simulink model "V1_DC_AC_PR_GF"  (R2022b)
settings: Solver=VariableStepAuto  StartTime=0.0  StopTime=.2  RelTol=1e-3
InitFcn:
  | %% Initialize twist parameters
  | source_V = 0;
  | Ts = 1e-7;
  | 
  | % set the PID parameters
  | Kp = 0.000215;
  | Ti = 7.5175e-5;
  | Td = 0.0;
  | N  = 0.0;
  | Kd = 0.0;
  | kp= 0.02;
  | kr = 4000;
  | fr = 10e3;
  | 
  | 
  | %Low side parameters
  | twist_low_side_L = 33e-6;
  | twist_low_side_rL = 20e-3; %Modified
  | twist_low_side_C = 47e-6 + 3*4.7e-6;
  | twist_low_side_C_electrolytic = 47e-6;
  | twist_low_side_C_ceramic = 3*4.7e-6;
  | twist_low_side_rC = 700e-3;
  | twist_low_side_rC_ceramic = 0;
  | twist_low_side_adc_R = 150e3+470;
  | 
  | %High side parameters
  | twist_high_side_C = 33e-6*4 + 4.7e-6*12;
  | twist_high_side_rC = 0.1;
  | twist_high_side_adc_R = 1/(1/2e6 + 1/2e6 + 1/(330e3+5.6e3));
  | twist_high_side_feeder_R = 47e3+4.7e3;
  | R_parallel = 1/(1/twist_high_side_adc_R + 1/twist_high_side_feeder_R);
  | tau_VCC = 0.204;
  | tau_desactive = 0.2;
  | twist_R_VCC = (tau_VCC/twist_high_side_C  - twist_high_side_rC)/(1-(tau_VCC/twist_high_side_C - twist_high_side_rC)/R_parallel);
  | 
  | %High side feeder current
  | %load('feeder_current.mat');
  | feeder_VHigh_min = 12;
  | feeder_VHigh_spacing = 6;
  | feeder_duty_min = 0.1;
  | feeder_duty_spacing = 0.4;
  | feeder_Vth_stop = 8.9;
  | feeder_Vth_start = 9.7;
  | feeder_current_upper_rate_limit = 0.386/(20e-3);
  | feeder_current_lower_rate_limit = -500;
  | 
  | %MOSFET parameters
  | twist_FET_Ron = 0.016;
  | twist_FET_Lon = 0;
  | twist_FET_Rd = 0.006;
  | twist_FET_Vf = 0.7;
  | twist_FET_Rs = 1e10;
  | twist_FET_Cs = inf;
  | twist_FET_Clow_Ron = 220e-3;
  | twist_FET_Clow_Rd = 45e-3; %Modified
  | twist_FET_Clow_Vf = 0.7; %Modified
  | 
  | 
  | %Schottky diode parameters
  | twist_shottky_Ron = 0.48; %Modified
  | twist_shottky_Vf = 0.28; %Modified
  | twist_shottky_Rs = 1e10;
  | twist_shottky_Cs = inf;
  | 
  | %PWM generation
  | twist_freq_switching = 200e3; %carry switching frequency
  | twist_period_switching = 1/twist_freq_switching; %carry switching period
  | twist_pwm_resolution = 100e-9; %resolution of the PWM generator - increasing it reduces simulation time
  | twist_duty_cycle_min = 0; %minimum duty cycle
  | twist_duty_cycle_max = 1; %maximum duty cycle
  | twist_dead_time = 200e-9; %duty cycle positive dead time
  | 
  | % Initialize times and frequencies
  | twist_freq_data_sampling = 20e3; %data sampling frequency
  | twist_data_sampling_period = 1/twist_freq_data_sampling; %data sampling delay
  | twist_data_acquisition_delay = 50e-9; %data acquisition at the peak of the carry
undefined symbols (not defined in the file): gcbh, sps_rtmsupport, twist_low_side_lC
libraries: spsSeriesRLCBranchLib x15, spsTriangleGeneratorLib x6, spsMosfetLib x6, spsCurrentMeasurementLib x4, spsVoltageMeasurementLib x4, spsControlledCurrentSourceLib x3, spsPLLLib x2, spsIdealSwitchLib x2, spsDiodeLib x2, spsACVoltageSourceLib x1, spsDCVoltageSourceLib x1, dspstat3 x1
(part 1 of 2)
settings Model: Creator=ABS_Lab  LastModifiedBy=ABS_Lab

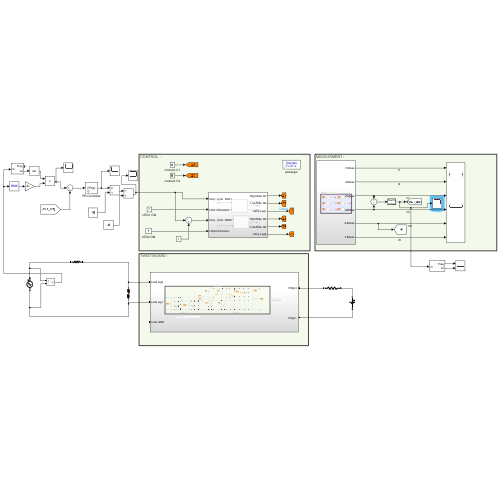
[thumbnail: Simulink's stored preview of the top-level diagram]
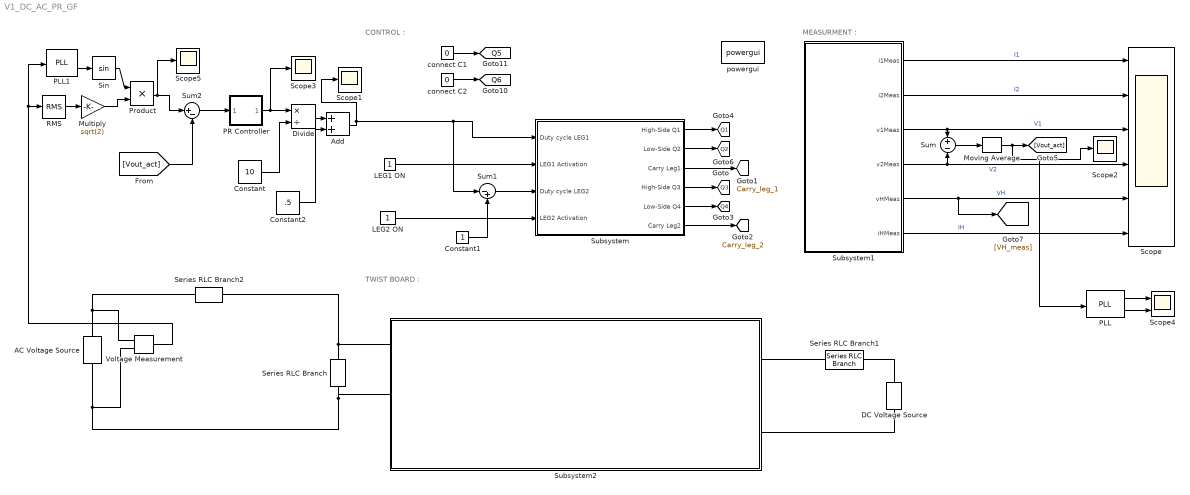
== system V1_DC_AC_PR_GF ==
  note: TWIST BOARD :
  note: CONTROL :
  note: MEASURMENT :
  AC Voltage Source : spsACVoltageSourceLib/AC Voltage Source  Amplitude=40  Phase=0  Frequency=50  SampleTime=0  Measurements=None  BusType=swing  Pref=10e3  Qref=0  Qmin=-inf  Qmax=+inf
  Add : Sum
  Constant : Constant  Value=10
  Constant1 : Constant
  Constant2 : Constant  Value=.5
  DC Voltage Source : spsDCVoltageSourceLib/DC Voltage Source  Amplitude=40  Measurements=None
  Divide : Product  Inputs=*/
  LEG1 ON : Constant
  LEG2 ON : Constant
  Moving Average : dspstat3/Moving Average  Method=Sliding window  ForgettingFactorPort=off  SpecifyWindowLength=on  WindowLength=15  OverlapLength=14  AllowArbitraryInputLength=off  ForgettingFactor=0.9  SimulateUsing=Code generation
  Multiply : Gain  Gain=sqrt(2)
  PLL : spsPLLLib/PLL  Fmin=45  Par_Init=[0, 50]  ParK=[180, 3200, 1]  TcD=1e-4  MaxRateChangeFreq=12  FilterCutOffFreq=25  Ts=0  AGC=on
      settings: LibrarySourceBlock=sps_lib/Control/PLL
  PLL1 : spsPLLLib/PLL  Fmin=45  Par_Init=[0, 50]  ParK=[180, 3200, 1]  TcD=1e-4  MaxRateChangeFreq=12  FilterCutOffFreq=25  Ts=0  AGC=on
      settings: LibrarySourceBlock=sps_lib/Control/PLL
  PR Controller : Subsystem  mask(PR Controller){kp=kp, kr=kr, f=fr}
      mask prompts: kp "Proportional Gain (kp)"; kr "Resonant Gain (kr)"; f "Resonant Frequency (Hz)"
      mask help:
      | This block implements a Proportional Resonant Controller using transfer function kr*s / s^2+(2*pi*f)^2
      | It allows user to set the proportional gain (kp), resonant gain (kr) and resonant frequency in (Hz).
      |
      | Developed by Rodney Tan
      | Version 1.0 (Oct 2022)
      mask Display: disp('PR(s)');
  Product : Product
  RMS : spsRMSLib/RMS  TrueRMS=on  Freq=60  RMSInit=120  Ts=0
  Scope : Scope  NumInputPorts=6
  Scope{1..3,5} (4 alike) : Scope
  Scope4 : Scope  NumInputPorts=2
  Series RLC Branch : spsSeriesRLCBranchLib/Series RLC Branch  LConnTagsString=__new0  RConnTagsString=__new0  BranchType=RL  Resistance=30  Inductance=100e-8  SetiL0=off  InitialCurrent=0  Capacitance=1e-6  Setx0=off  InitialVoltage=0  Measurements=None
  Series RLC Branch1 : spsSeriesRLCBranchLib/Series RLC Branch  LConnTagsString=__new0  RConnTagsString=__new0  BranchType=R  Resistance=100e-3  Inductance=1e-3  SetiL0=off  InitialCurrent=0  Capacitance=1e-6  Setx0=off  InitialVoltage=0  Measurements=None
  Series RLC Branch2 : spsSeriesRLCBranchLib/Series RLC Branch  LConnTagsString=__new0  RConnTagsString=__new0  BranchType=R  Resistance=.01  Inductance=100e-8  SetiL0=off  InitialCurrent=0  Capacitance=1e-6  Setx0=off  InitialVoltage=0  Measurements=None
  Sin : Trigonometry
  Subsystem : Subsystem
  Subsystem1 : Subsystem
  Subsystem2 : Subsystem
  Sum : Sum  Inputs=+-
  Sum1 : Sum  Inputs=|-+
  Sum2 : Sum  Inputs=|+-
  Voltage Measurement : spsVoltageMeasurementLib/Voltage Measurement  PhasorSimulation=off  OutputType=Complex  PSBequivalent=0
  connect C1 : Constant  Value=0
  connect C2 : Constant  Value=0
  powergui : sps_lib/powergui  Priority=1  SimulationMode=Discrete  SampleTime=Ts  frequency=60  Iterations=50  frequencyindice=0  Pbase=100e6  ErrMax=1e-4  UnitsV=kV  UnitsW=MW  buscounter=0  FunctionMessages=off  echomessages=off  EnableUseOfTLC=off  CurrentSourceSwitches=off  DisableSnubberDevices=off  DisableRonSwitches=off  DisableVfSwitches=off  DisplayEquations=off  AutomaticDiscreteSolvers=off  SolverType=Tustin/Backward Euler (TBE)  Interpol=off  ExternalGateDelay=off  methode=off  Ts=100  x0status=blocks  SPID=on  SwTol=0  HookPort=off  NonlinearTolerance=1e-4  nMaxIteration=100  ContinueOnMaxIteration=off  RestoreLinks=warning  ResistiveCurrentMeasurement=off  Frange=[0:2:500]  Ylog=off  Xlog=on  ShowGrid=off  save=off  variable=ZData  structure=0  ZoomFFT=off  StartTime=0.0  cycles=1  DisplayStyle=1  fundamental=60  FreqAxis=off  MaxFrequency=1000  frequencyindicesteady=1  RmsSteady=1  display=off
  tag scope: Carry_leg_1=global, Carry_leg_2=global, Q1=global, Q2=global, Q3=global, Q4=global, Q5=global, Q6=global
  wires:
  LEG1 ON/1 -> Subsystem/2(LEG1 Activation)
  LEG2 ON/1 -> Subsystem/4("LEG2 Activation ")
  Subsystem/3(Carry Leg1) -> [Carry_leg_1]
  Subsystem/6(Carry Leg2) -> [Carry_leg_2]
  Subsystem1/6(iHMeas) -> Scope/6  "IH"
  Subsystem1/5(vHMeas) -> [VH_meas], Scope/5  "VH"
  Subsystem1/3(v1Meas) -> Sum/1, Scope/3  "V1"
  Subsystem1/4(v2Meas) -> Sum/2, Scope/4  "V2"
  Subsystem1/2(i2Meas) -> Scope/2  "I2"
  connect C1/1 -> [Q5]
  connect C2/1 -> [Q6]
  Subsystem1/1(i1Meas) -> Scope/1  "I1"
  Constant1/1 -> Sum1/2
  Sum1/1 -> Subsystem/3(Duty cycle LEG2)
  Sum2/1 -> PR Controller/1(In1)
  [Vout_act] -> Sum2/2
  Moving Average/1 -> PLL/1, Scope2/1, [Vout_act]
  Sum/1 -> Moving Average/1
  Subsystem/1(High-Side Q1) -> [Q1]
  Subsystem/2(Low-Side Q2) -> [Q2]
  Subsystem/4(High-Side Q3) -> [Q3]
  Subsystem/5(Low-Side Q4) -> [Q4]
  PR Controller/1(Out1) -> Scope3/1, Divide/1
  Constant/1 -> Divide/2
  Divide/1 -> Add/1
  Constant2/1 -> Add/2
  Add/1 -> Sum1/1, Subsystem/1(Duty cycle LEG1), Scope1/1
  PLL/1 -> Scope4/1
  PLL/2 -> Scope4/2
  Voltage Measurement/1 -> RMS/1, PLL1/1
  PLL1/2 -> Sin/1
  RMS/1 -> Multiply/1
  Product/1 -> Scope5/1, Sum2/1
  Sin/1 -> Product/1
  Multiply/1 -> Product/2
  connections:
  Series RLC Branch/LConn1 -- Series RLC Branch2/LConn1 -- Subsystem2/LConn1
  DC Voltage Source/LConn1 -- Subsystem2/RConn2
  Series RLC Branch1/LConn1 -- Subsystem2/RConn1
  DC Voltage Source/RConn1 -- Series RLC Branch1/RConn1
  Subsystem2/LConn2 -- Voltage Measurement/LConn2 -- AC Voltage Source/LConn1 -- Series RLC Branch/RConn1
  Voltage Measurement/LConn1 -- Series RLC Branch2/RConn1 -- AC Voltage Source/RConn1

== system V1_DC_AC_PR_GF/PR Controller ==
  In1 : Inport
  Gain : Gain  Gain=kp
  Gain1 : Gain  Gain=kr
  Saturation : Saturate  UpperLimit=40  LowerLimit=-40
  Sum1 : Sum  Inputs=|++
  Transfer Fcn1 : TransferFcn  Numerator=[1 0]  Denominator=[1 0 (2*pi*fr)^2]
  Out1 : Outport
  wires:
  Gain1/1 -> Transfer Fcn1/1
  Transfer Fcn1/1 -> Sum1/2
  In1/1 -> Gain1/1, Gain/1
  Gain/1 -> Sum1/1
  Sum1/1 -> Saturation/1
  Saturation/1 -> Out1/1

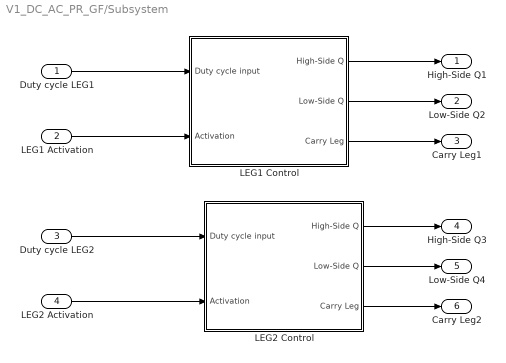
== system V1_DC_AC_PR_GF/Subsystem ==
  Duty cycle LEG1 : Inport
  LEG1 Activation : Inport  Port=2
  Duty cycle LEG2 : Inport  Port=3
  "LEG2 Activation " : Inport  Port=4
  "LEG1 Control " : Subsystem
  LEG2 Control : Subsystem
  High-Side Q1 : Outport
  Low-Side Q2 : Outport  Port=2
  Carry Leg1 : Outport  Port=3
  High-Side Q3 : Outport  Port=4
  Low-Side Q4 : Outport  Port=5
  Carry Leg2 : Outport  Port=6
  wires:
  "LEG1 Control "/3(Carry Leg) -> Carry Leg1/1
  LEG2 Control/1(High-Side Q) -> High-Side Q3/1
  Duty cycle LEG1/1 -> "LEG1 Control "/1(Duty cycle input)
  Duty cycle LEG2/1 -> LEG2 Control/1(Duty cycle input)
  LEG1 Activation/1 -> "LEG1 Control "/2(Activation)
  LEG2 Control/2(Low-Side Q) -> Low-Side Q4/1
  "LEG2 Activation "/1 -> LEG2 Control/2(Activation)
  LEG2 Control/3(Carry Leg) -> Carry Leg2/1
  "LEG1 Control "/1(High-Side Q) -> High-Side Q1/1
  "LEG1 Control "/2(Low-Side Q) -> Low-Side Q2/1

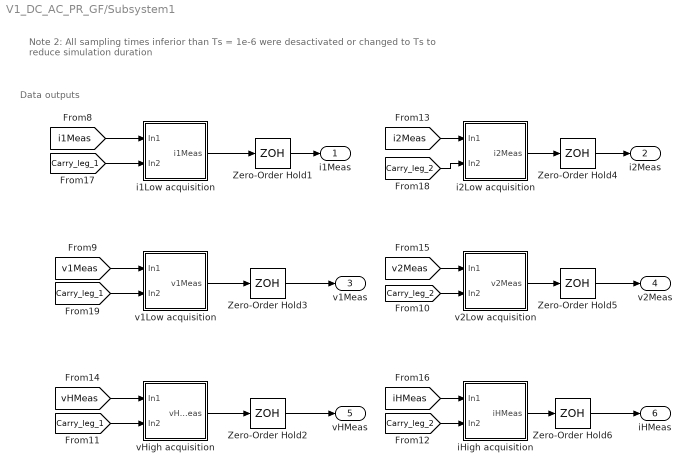
== system V1_DC_AC_PR_GF/Subsystem1 ==
  note: Note 2:
      | All sampling times inferior than Ts = 1e-6 were desactivated or changed to Ts to reduce simulation duration
  note: Data outputs
  Zero-Order Hold{1..6} (6 alike) : ZeroOrderHold  SampleTime=twist_data_sampling_period
  i1Low acquisition : Subsystem
  i2Low acquisition : Subsystem
  iHigh acquisition : Subsystem
  v1Low acquisition : Subsystem
  v2Low acquisition : Subsystem
  vHigh acquisition : Subsystem
  i1Meas : Outport
  i2Meas : Outport  Port=2
  v1Meas : Outport  Port=3
  v2Meas : Outport  Port=4
  vHMeas : Outport  Port=5
  iHMeas : Outport  Port=6
  wires:
  i1Low acquisition/1(i1Meas) -> Zero-Order Hold1/1
  [v1Meas] -> v1Low acquisition/1(In1)
  [v2Meas] -> v2Low acquisition/1(In1)
  [Carry_leg_2] -> v2Low acquisition/2(In2)
  [i2Meas] -> i2Low acquisition/1(In1)
  [Carry_leg_2] -> i2Low acquisition/2(In2)
  [vHMeas] -> vHigh acquisition/1(In1)
  [Carry_leg_1] -> vHigh acquisition/2(In2)
  [Carry_leg_2] -> iHigh acquisition/2(In2)
  [Carry_leg_1] -> v1Low acquisition/2(In2)
  [Carry_leg_1] -> i1Low acquisition/2(In2)
  [iHMeas] -> iHigh acquisition/1(In1)
  [i1Meas] -> i1Low acquisition/1(In1)
  Zero-Order Hold5/1 -> v2Meas/1
  Zero-Order Hold3/1 -> v1Meas/1
  Zero-Order Hold1/1 -> i1Meas/1
  i2Low acquisition/1(i2Meas) -> Zero-Order Hold4/1
  Zero-Order Hold4/1 -> i2Meas/1
  v1Low acquisition/1(v1Meas) -> Zero-Order Hold3/1
  v2Low acquisition/1(v2Meas) -> Zero-Order Hold5/1
  vHigh acquisition/1(vHMeas) -> Zero-Order Hold2/1
  Zero-Order Hold2/1 -> vHMeas/1
  iHigh acquisition/1(iHMeas) -> Zero-Order Hold6/1
  Zero-Order Hold6/1 -> iHMeas/1

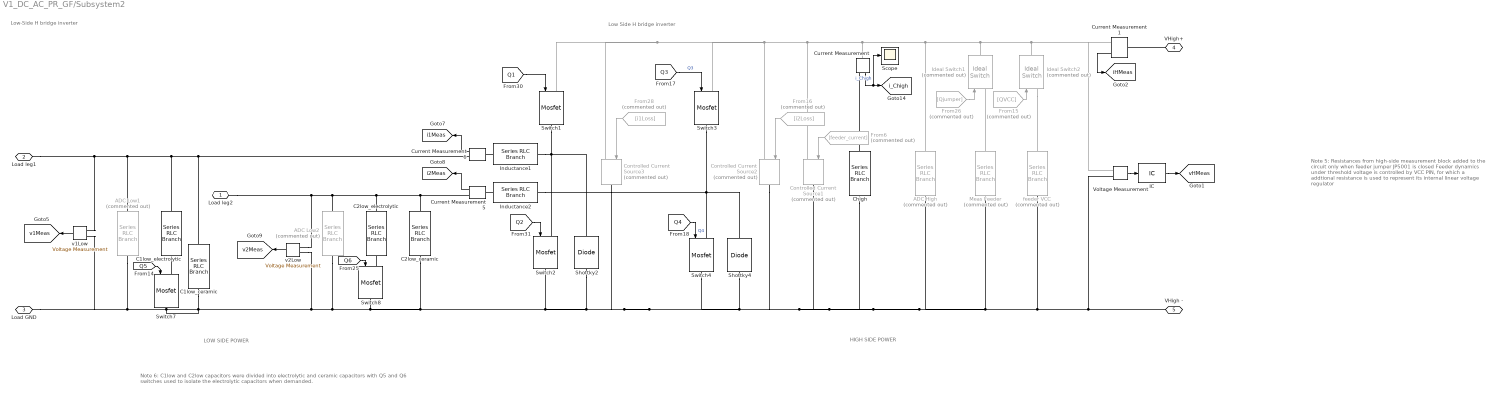
== system V1_DC_AC_PR_GF/Subsystem2 ==
  note: Note 5:
      |
      | Resistances from high-side measurement block added to the circuit only when feeder jumper JP5001 is closed
      |
      | Feeder dynamics under threshold voltage is controlled by VCC PIN, for which a addtional resistance is used to represent its internal linear voltage regulator
  note: Note 6:
      | C1low and C2low capacitors were divided into electrolytic and ceramic capacitors with Q5 and Q6 switches used to isolate the electrolytic capacitors when demanded.
  note: Low Side H bridge inverter
  note: LOW SIDE POWER
  note: HIGH SIDE POWER
  note: Low-Side H bridge inverter
  ADC High : spsSeriesRLCBranchLib/Series RLC Branch  Commented=on  LConnTagsString=__new0  RConnTagsString=__new0  BranchType=R  Resistance=twist_high_side_adc_R  Inductance=twist_low_side_L  SetiL0=off  InitialCurrent=0  Capacitance=1e-6  Setx0=off  InitialVoltage=0  Measurements=None
  ADC Low1 : spsSeriesRLCBranchLib/Series RLC Branch  Commented=on  LConnTagsString=__new0  RConnTagsString=__new0  BranchType=R  Resistance=twist_low_side_adc_R  Inductance=twist_low_side_L  SetiL0=off  InitialCurrent=0  Capacitance=1e-6  Setx0=off  InitialVoltage=0  Measurements=Branch voltage
  ADC Low2 : spsSeriesRLCBranchLib/Series RLC Branch  Commented=on  LConnTagsString=__new0  RConnTagsString=__new0  BranchType=R  Resistance=twist_low_side_adc_R  Inductance=twist_low_side_L  SetiL0=off  InitialCurrent=0  Capacitance=1e-6  Setx0=off  InitialVoltage=0  Measurements=Branch voltage
  C1low_ceramic : spsSeriesRLCBranchLib/Series RLC Branch  LConnTagsString=__new0  RConnTagsString=__new0  BranchType=C  Resistance=twist_low_side_rC  Inductance=1e-3  SetiL0=off  InitialCurrent=0  Capacitance=twist_low_side_C_ceramic  Setx0=off  InitialVoltage=source_V  Measurements=None
  C1low_electrolytic : spsSeriesRLCBranchLib/Series RLC Branch  LConnTagsString=__new0  RConnTagsString=__new0  BranchType=RC  Resistance=twist_low_side_rC  Inductance=twist_low_side_lC  SetiL0=off  InitialCurrent=0  Capacitance=twist_low_side_C_electrolytic  Setx0=off  InitialVoltage=source_V  Measurements=None
  C2low_ceramic : spsSeriesRLCBranchLib/Series RLC Branch  LConnTagsString=__new0  RConnTagsString=__new0  BranchType=C  Resistance=twist_low_side_rC  Inductance=1e-3  SetiL0=off  InitialCurrent=0  Capacitance=twist_low_side_C_ceramic  Setx0=off  InitialVoltage=source_V  Measurements=None
  C2low_electrolytic : spsSeriesRLCBranchLib/Series RLC Branch  LConnTagsString=__new0  RConnTagsString=__new0  BranchType=RC  Resistance=twist_low_side_rC  Inductance=twist_low_side_lC  SetiL0=off  InitialCurrent=0  Capacitance=twist_low_side_C_electrolytic  Setx0=off  InitialVoltage=source_V  Measurements=None
  Chigh : spsSeriesRLCBranchLib/Series RLC Branch  LConnTagsString=__new0  RConnTagsString=__new0  BranchType=RC  Resistance=twist_high_side_rC  Inductance=1e-3  SetiL0=off  InitialCurrent=0  Capacitance=twist_high_side_C  Setx0=on  InitialVoltage=source_V  Measurements=None
  Controlled Current Source1 : spsControlledCurrentSourceLib/Controlled Current Source  Commented=on  Initialize=on  Source_Type=AC  Amplitude=0  Phase=0  Frequency=0  Measurements=None
  Controlled Current Source2 : spsControlledCurrentSourceLib/Controlled Current Source  Commented=on  Initialize=on  Source_Type=AC  Amplitude=0  Phase=0  Frequency=0  Measurements=None
  Controlled Current Source3 : spsControlledCurrentSourceLib/Controlled Current Source  Commented=on  Initialize=on  Source_Type=AC  Amplitude=0  Phase=0  Frequency=0  Measurements=None
  Current Measurement{,1,5..6} (4 alike) : spsCurrentMeasurementLib/Current Measurement  PhasorSimulation=off  OutputType=Complex  PSBequivalent=0
  From15 : From  Commented=on  GotoTag=QVCC
  From16 : From  Commented=on  GotoTag=i2Loss
  From26 : From  Commented=on  GotoTag=Qjumper
  From28 : From  Commented=on  GotoTag=i1Loss
  From6 : From  Commented=on  GotoTag=feeder_current
  IC : InitialCondition  Value=source_V
  Ideal Switch1 : spsIdealSwitchLib/Ideal Switch  Commented=on  Ron=0.001  Lon=0  IC=0  Rs=1e5  Cs=inf  Measurements=off
  Ideal Switch2 : spsIdealSwitchLib/Ideal Switch  Commented=on  Ron=0.001  Lon=0  IC=0  Rs=1e5  Cs=inf  Measurements=off
  Inductance1 : spsSeriesRLCBranchLib/Series RLC Branch  LConnTagsString=__new0  RConnTagsString=__new0  BranchType=RL  Resistance=twist_low_side_rL  Inductance=twist_low_side_L  SetiL0=off  InitialCurrent=0  Capacitance=1e-6  Setx0=off  InitialVoltage=0  Measurements=None
  Inductance2 : spsSeriesRLCBranchLib/Series RLC Branch  LConnTagsString=__new0  RConnTagsString=__new0  BranchType=RL  Resistance=twist_low_side_rL  Inductance=twist_low_side_L  SetiL0=off  InitialCurrent=0  Capacitance=1e-6  Setx0=off  InitialVoltage=0  Measurements=None
  Meas Feeder : spsSeriesRLCBranchLib/Series RLC Branch  Commented=on  LConnTagsString=__new0  RConnTagsString=__new0  BranchType=R  Resistance=twist_high_side_feeder_R  Inductance=twist_low_side_L  SetiL0=off  InitialCurrent=0  Capacitance=1e-6  Setx0=off  InitialVoltage=0  Measurements=None
  Scope : Scope
  Shottky2 : spsDiodeLib/Diode  Ron=twist_shottky_Ron  Lon=0  Vf=twist_shottky_Vf  IC=0  UseSnubber=0  Rs=twist_shottky_Rs  Cs=twist_shottky_Cs  Measurements=off
  Shottky4 : spsDiodeLib/Diode  Ron=twist_shottky_Ron  Lon=0  Vf=twist_shottky_Vf  IC=0  UseSnubber=0  Rs=twist_shottky_Rs  Cs=twist_shottky_Cs  Measurements=off
  Switch{1..4} (4 alike) : spsMosfetLib/Mosfet  Ron=twist_FET_Ron  Lon=0  Rd=twist_FET_Rd  Vfd=twist_FET_Vf  IC=0  Rs=twist_FET_Rs  Cs=twist_FET_Cs  Measurements=off
  Switch7 : spsMosfetLib/Mosfet  Ron=twist_FET_Clow_Ron  Lon=0  Rd=twist_FET_Clow_Ron  Vfd=0  IC=0  Rs=twist_FET_Rs  Cs=twist_FET_Cs  Measurements=off
  Switch8 : spsMosfetLib/Mosfet  Ron=twist_FET_Clow_Ron  Lon=0  Rd=twist_FET_Clow_Ron  Vfd=0  IC=0  Rs=twist_FET_Rs  Cs=twist_FET_Cs  Measurements=off
  Voltage Measurement : spsVoltageMeasurementLib/Voltage Measurement  PhasorSimulation=off  OutputType=Complex  PSBequivalent=0
  feeder VCC : spsSeriesRLCBranchLib/Series RLC Branch  Commented=on  LConnTagsString=__new0  RConnTagsString=__new0  BranchType=R  Resistance=twist_R_VCC  Inductance=twist_low_side_L  SetiL0=off  InitialCurrent=0  Capacitance=1e-6  Setx0=off  InitialVoltage=0  Measurements=None
  v1Low : spsVoltageMeasurementLib/Voltage Measurement  PhasorSimulation=off  OutputType=Complex  PSBequivalent=0
  v2Low : spsVoltageMeasurementLib/Voltage Measurement  PhasorSimulation=off  OutputType=Complex  PSBequivalent=0
  Load leg2 : PMIOPort  Side=Left
  Load leg1 : PMIOPort  Port=2  Side=Left
  Load GND : PMIOPort  Port=3  Side=Left
  VHigh+ : PMIOPort  Port=4  Side=Right
  VHigh - : PMIOPort  Port=5  Side=Right
  tag scope: i1Meas=global, i2Meas=global, iHMeas=global, i_Chigh=global, v1Meas=global, v2Meas=global, vHMeas=global
  wires:
  From28/1 -> Controlled Current Source3/1
  From6/1 -> Controlled Current Source1/1
  Current Measurement5/1 -> [i2Meas]
  Current Measurement1/1 -> [iHMeas]
  Current Measurement6/1 -> [i1Meas]
  Current Measurement/1 -> [i_Chigh], Scope/1  "i_Chigh"
  [Q1] -> Switch1/1
  [Q3] -> Switch3/1  "Q3"
  IC/1 -> [vHMeas]
  From15/1 -> Ideal Switch2/1
  [Q5] -> Switch7/1
  [Q4] -> Switch4/1  "Q4"
  Voltage Measurement/1 -> IC/1
  v2Low/1 -> [v2Meas]
  [Q6] -> Switch8/1
  From16/1 -> Controlled Current Source2/1
  [Q2] -> Switch2/1
  v1Low/1 -> [v1Meas]
  From26/1 -> Ideal Switch1/1
  connections:
  Inductance2/LConn1 -- Current Measurement5/LConn1
  Current Measurement/RConn1 -- Chigh/LConn1
  VHigh+/RConn1 -- Current Measurement1/LConn1
  Ideal Switch2/LConn1 -- feeder VCC/LConn1
  Meas Feeder/LConn1 -- Ideal Switch1/LConn1
  Load leg1/RConn1 -- ADC Low1/LConn1 -- C1low_electrolytic/LConn1 -- Current Measurement6/RConn1 -- C1low_ceramic/LConn1 -- v1Low/LConn1
  Load leg2/RConn1 -- Current Measurement5/RConn1 -- C2low_ceramic/LConn1 -- C2low_electrolytic/LConn1 -- ADC Low2/LConn1 -- v2Low/LConn1
  Switch3/RConn1 -- Switch4/LConn1 -- Inductance2/RConn1 -- Shottky4/RConn1
  Switch7/LConn1 -- C1low_electrolytic/RConn1
  Ideal Switch1/RConn1 -- Ideal Switch2/RConn1 -- Current Measurement1/RConn1 -- Voltage Measurement/LConn1 -- ADC High/LConn1 -- Current Measurement/LConn1 -- Controlled Current Source1/LConn1 -- Controlled Current Source2/LConn1 -- Switch3/LConn1 -- Switch1/LConn1 -- Controlled Current Source3/LConn1
  Current Measurement6/LConn1 -- Inductance1/LConn1
  Switch8/LConn1 -- C2low_electrolytic/RConn1
  Shottky2/RConn1 -- Inductance1/RConn1 -- Switch1/RConn1 -- Switch2/LConn1
  VHigh -/RConn1 -- Shottky2/LConn1 -- C2low_ceramic/RConn1 -- Switch8/RConn1 -- ADC Low2/RConn1 -- C1low_ceramic/RConn1 -- Switch7/RConn1 -- ADC Low1/RConn1 -- v1Low/LConn2 -- Load GND/RConn1 -- v2Low/LConn2 -- Switch2/RConn1 -- Controlled Current Source3/RConn1 -- Switch4/RConn1 -- Shottky4/LConn1 -- Controlled Current Source2/RConn1 -- Controlled Current Source1/RConn1 -- Chigh/RConn1 -- ADC High/RConn1 -- Meas Feeder/RConn1 -- feeder VCC/RConn1 -- Voltage Measurement/LConn2

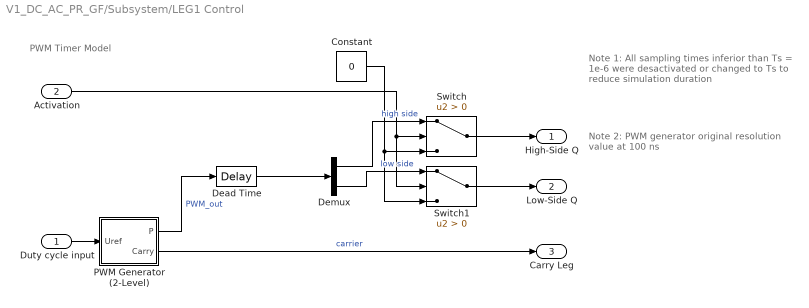
== system V1_DC_AC_PR_GF/Subsystem/LEG1 Control  ==
  note: Note 1:
      | All sampling times inferior than Ts = 1e-6 were desactivated or changed to Ts to reduce simulation duration
  note: PWM Timer Model
  note: Note 2:
      | PWM generator original resolution value at 100 ns
  Duty cycle input : Inport
  Activation : Inport  Port=2
  Constant : Constant  Value=0
  Dead Time : TransportDelay  DelayTime=twist_dead_time
  Demux : Demux  Outputs=2
  PWM Generator (2-Level) : Subsystem  AncestorBlock=|  DialogController=POWERSYS.PowerSysDialog  LoadFcn=sps_rtmsupport('LoadFcn', gcbh);  StartFcn=sps_rtmsupport('StartFcn', gcbh);  StopFcn=sps_rtmsupport('StopFcn', gcbh);  BlockChoice=InternalUref  mask(PWM Generator (2-Level)){ModulatorType=Single-phase half-bridge (2 pulses), ModulatorMode=Unsynchronized, Fc=twist_freq_switching, Pc=0, nF=27, MinMax=[0 1], SamplingTechnique=Symmetrical regular (single edge), ModulatingSignals=off, m=0.8, Freq=60, Phase=0, Ts=Ts, ShowCarrierOutport=off}
      | spsPWMGenerator2LevelLib/PWM Generator
      | (2-Level)
      mask prompts: ModulatorType "Generator type:"; ModulatorMode "Mode of operation:"; Fc "Frequency (Hz):"; Pc "Initial phase (degrees):"; nF "Switching ratio (carrier frequency / output frequency):"; MinMax "Minimum and maximum values: [ Min  Max ]"; SamplingTechnique "Sampling technique:"; ModulatingSignals "Internal generation of reference signal"; m "Modulation index:"; Freq "Frequency (Hz):"; Phase "Phase (degrees):"; Ts "Sample time (s):"; ShowCarrierOutport "Show measurement port"
      mask help:
      | Generate pulses for PWM-controlled 2-Level converter, using carrier-based two-level PWM method. The block can control switching devices of single-phase half-bridge, single-phase full-bridge (unipolar or bipolar modulation) or three-phase bridge.
      |
      | When the Synchronized mode of operation is selected, a second input is added to the block, and the internal generation of modulating signal is disabled. Use input 2 (wt) to synchronize the carrier.
      mask init:
      | sps = powericon('PWMGenerator2LevelInit',gcb,ModulatorType,SamplingTechnique,ModulatorMode,nF,Fc,MinMax,Pc,ShowCarrierOutport,ModulatingSignals,m,Freq,Phase,Ts);
      settings: CopyFcn=sps_rtmsupport('CopyFcn', gcbh);  DeleteFcn=sps_rtmsupport('DeleteFcn', gcbh);  UndoDeleteFcn=sps_rtmsupport('UndoDeleteFcn', gcbh);  ModelCloseFcn=sps_rtmsupport('ModelCloseFcn', gcbh);  PreSaveFcn=sps_rtmsupport('PreSaveFcn', gcbh);  PostSaveFcn=sps_rtmsupport('PostSaveFcn', gcbh);  NameChangeFcn=sps_rtmsupport('NameChangeFcn', gcbh);  PreCopyFcn=sps_rtmsupport('PreCopyFcn', gcbh);  OpenFcn="sps_rtmsupport('OpenFcn', gcbh, [1   2   7   8  13]);"  CloseFcn=sps_rtmsupport('CloseFcn', gcbh);  PreDeleteFcn=sps_rtmsupport('PreDeleteFcn', gcbh);
      settings: LibrarySourceBlock=|
      | spsPWMGenerator2LevelLib/PWM Generator
      | (2-Level)
      mask Help: helpview(psbhelp);
      mask TypeOptions ModulatorType: Single-phase half-bridge (2 pulses) | Single-phase full-bridge (4 pulses) | Single-phase full-bridge - Bipolar modulation (4 pulses) | Three-phase bridge (6 pulses)
      mask TypeOptions ModulatorMode: Synchronized | Unsynchronized
      mask Callback ModulatorMode: powericon('PWMGenerator2LevelCback',gcb);
      mask TypeOptions SamplingTechnique: Natural | Asymmetrical regular (double edge) | Symmetrical regular (single edge)
      mask Callback ModulatingSignals: powericon('PWMGenerator2LevelCback',gcb);
      mask DialogControl Container3 Prompt: Carrier
      mask DialogControl ModulatingSignalParameters Prompt: Reference signal
  Switch : Switch  Criteria=u2 > Threshold  SaturateOnIntegerOverflow=off  InputSameDT=off
  Switch1 : Switch  Criteria=u2 > Threshold  SaturateOnIntegerOverflow=off  InputSameDT=off
  High-Side Q : Outport
  Low-Side Q : Outport  Port=2
  Carry Leg : Outport  Port=3
  wires:
  Switch1/1 -> Low-Side Q/1
  PWM Generator (2-Level)/1(P) -> Dead Time/1  "PWM_out"
  Demux/1 -> Switch/1  "high side"
  PWM Generator (2-Level)/2(Carry) -> Carry Leg/1  "carrier"
  Activation/1 -> Switch/2, Switch1/2
  Switch/1 -> High-Side Q/1
  Demux/2 -> Switch1/1  "low side"
  Duty cycle input/1 -> PWM Generator (2-Level)/1(Uref)
  Constant/1 -> Switch1/3, Switch/3
  Dead Time/1 -> Demux/1

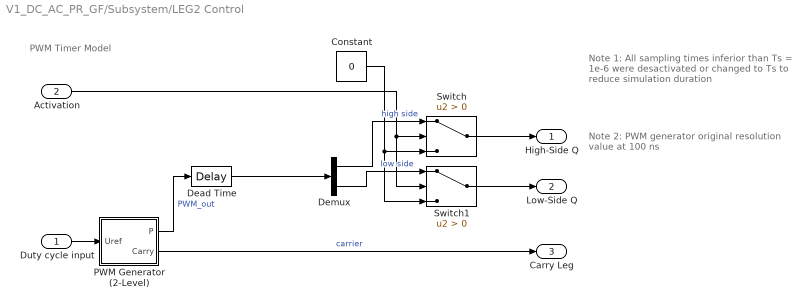
== system V1_DC_AC_PR_GF/Subsystem/LEG2 Control ==
  note: Note 2:
      | PWM generator original resolution value at 100 ns
  note: PWM Timer Model
  note: Note 1:
      | All sampling times inferior than Ts = 1e-6 were desactivated or changed to Ts to reduce simulation duration
  Duty cycle input : Inport
  Activation : Inport  Port=2
  Constant : Constant  Value=0
  Dead Time : TransportDelay  DelayTime=twist_dead_time
  Demux : Demux  Outputs=2
  PWM Generator (2-Level) : Subsystem  AncestorBlock=|  DialogController=POWERSYS.PowerSysDialog  LoadFcn=sps_rtmsupport('LoadFcn', gcbh);  StartFcn=sps_rtmsupport('StartFcn', gcbh);  StopFcn=sps_rtmsupport('StopFcn', gcbh);  BlockChoice=InternalUref  mask(PWM Generator (2-Level)){ModulatorType=Single-phase half-bridge (2 pulses), ModulatorMode=Unsynchronized, Fc=twist_freq_switching, Pc=0, nF=27, MinMax=[0 1], SamplingTechnique=Symmetrical regular (single edge), ModulatingSignals=off, m=0.8, Freq=60, Phase=0, Ts=Ts, ShowCarrierOutport=off}
      | spsPWMGenerator2LevelLib/PWM Generator
      | (2-Level)
      mask prompts: ModulatorType "Generator type:"; ModulatorMode "Mode of operation:"; Fc "Frequency (Hz):"; Pc "Initial phase (degrees):"; nF "Switching ratio (carrier frequency / output frequency):"; MinMax "Minimum and maximum values: [ Min  Max ]"; SamplingTechnique "Sampling technique:"; ModulatingSignals "Internal generation of reference signal"; m "Modulation index:"; Freq "Frequency (Hz):"; Phase "Phase (degrees):"; Ts "Sample time (s):"; ShowCarrierOutport "Show measurement port"
      mask help:
      | Generate pulses for PWM-controlled 2-Level converter, using carrier-based two-level PWM method. The block can control switching devices of single-phase half-bridge, single-phase full-bridge (unipolar or bipolar modulation) or three-phase bridge.
      |
      | When the Synchronized mode of operation is selected, a second input is added to the block, and the internal generation of modulating signal is disabled. Use input 2 (wt) to synchronize the carrier.
      mask init:
      | sps = powericon('PWMGenerator2LevelInit',gcb,ModulatorType,SamplingTechnique,ModulatorMode,nF,Fc,MinMax,Pc,ShowCarrierOutport,ModulatingSignals,m,Freq,Phase,Ts);
      settings: CopyFcn=sps_rtmsupport('CopyFcn', gcbh);  DeleteFcn=sps_rtmsupport('DeleteFcn', gcbh);  UndoDeleteFcn=sps_rtmsupport('UndoDeleteFcn', gcbh);  ModelCloseFcn=sps_rtmsupport('ModelCloseFcn', gcbh);  PreSaveFcn=sps_rtmsupport('PreSaveFcn', gcbh);  PostSaveFcn=sps_rtmsupport('PostSaveFcn', gcbh);  NameChangeFcn=sps_rtmsupport('NameChangeFcn', gcbh);  PreCopyFcn=sps_rtmsupport('PreCopyFcn', gcbh);  OpenFcn="sps_rtmsupport('OpenFcn', gcbh, [1   2   7   8  13]);"  CloseFcn=sps_rtmsupport('CloseFcn', gcbh);  PreDeleteFcn=sps_rtmsupport('PreDeleteFcn', gcbh);
      settings: LibrarySourceBlock=|
      | spsPWMGenerator2LevelLib/PWM Generator
      | (2-Level)
      mask Help: helpview(psbhelp);
      mask TypeOptions ModulatorType: Single-phase half-bridge (2 pulses) | Single-phase full-bridge (4 pulses) | Single-phase full-bridge - Bipolar modulation (4 pulses) | Three-phase bridge (6 pulses)
      mask TypeOptions ModulatorMode: Synchronized | Unsynchronized
      mask Callback ModulatorMode: powericon('PWMGenerator2LevelCback',gcb);
      mask TypeOptions SamplingTechnique: Natural | Asymmetrical regular (double edge) | Symmetrical regular (single edge)
      mask Callback ModulatingSignals: powericon('PWMGenerator2LevelCback',gcb);
      mask DialogControl Container3 Prompt: Carrier
      mask DialogControl ModulatingSignalParameters Prompt: Reference signal
  Switch : Switch  Criteria=u2 > Threshold  SaturateOnIntegerOverflow=off  InputSameDT=off
  Switch1 : Switch  Criteria=u2 > Threshold  SaturateOnIntegerOverflow=off  InputSameDT=off
  High-Side Q : Outport
  Low-Side Q : Outport  Port=2
  Carry Leg : Outport  Port=3
  wires:
  Constant/1 -> Switch/3, Switch1/3
  Duty cycle input/1 -> PWM Generator (2-Level)/1(Uref)
  Demux/2 -> Switch1/1  "low side"
  Activation/1 -> Switch1/2, Switch/2
  PWM Generator (2-Level)/2(Carry) -> Carry Leg/1  "carrier"
  Demux/1 -> Switch/1  "high side"
  PWM Generator (2-Level)/1(P) -> Dead Time/1  "PWM_out"
  Switch/1 -> High-Side Q/1
  Switch1/1 -> Low-Side Q/1
  Dead Time/1 -> Demux/1

== system V1_DC_AC_PR_GF/Subsystem1/i1Low acquisition ==
  In1 : Inport
  In2 : Inport  Port=2
  If : If  IfExpression=u1 > 0.99  ShowElse=off
  If Action Subsystem : Subsystem  TreatAsAtomicUnit=on
  Scope : Scope  NumInputPorts=3
  i1Meas : Outport
  wires:
  If Action Subsystem/1(Out1) -> Scope/1, i1Meas/1  "Data_Carry"
  In1/1 -> Scope/2, If Action Subsystem/1(In1)  "Data"
  If/1 -> If Action Subsystem/Action
  In2/1 -> If/1, Scope/3  "Carry"

== system V1_DC_AC_PR_GF/Subsystem1/i2Low acquisition ==
  In1 : Inport
  In2 : Inport  Port=2
  If : If  IfExpression=u1 > 0.99  ShowElse=off
  If Action Subsystem : Subsystem  TreatAsAtomicUnit=on
  Scope : Scope  NumInputPorts=3
  i2Meas : Outport
  wires:
  If Action Subsystem/1(Out1) -> Scope/1, i2Meas/1  "Data_Carry"
  In1/1 -> Scope/2, If Action Subsystem/1(In1)  "Data"
  If/1 -> If Action Subsystem/Action
  In2/1 -> If/1, Scope/3  "Carry"

== system V1_DC_AC_PR_GF/Subsystem1/iHigh acquisition ==
  In1 : Inport
  In2 : Inport  Port=2
  If : If  IfExpression=u1 > 0.99  ShowElse=off
  If Action Subsystem : Subsystem  TreatAsAtomicUnit=on
  Scope : Scope  NumInputPorts=3
  iHMeas : Outport
  wires:
  If Action Subsystem/1(Out1) -> Scope/1, iHMeas/1  "Data_Carry"
  In1/1 -> Scope/2, If Action Subsystem/1(In1)  "Data"
  If/1 -> If Action Subsystem/Action
  In2/1 -> If/1, Scope/3  "Carry"

== system V1_DC_AC_PR_GF/Subsystem1/v1Low acquisition ==
  In1 : Inport
  In2 : Inport  Port=2
  If : If  IfExpression=u1 > 0.99  ShowElse=off
  If Action Subsystem : Subsystem  TreatAsAtomicUnit=on
  Scope : Scope  NumInputPorts=3
  v1Meas : Outport
  wires:
  If Action Subsystem/1(Out1) -> Scope/1, v1Meas/1  "Data_Carry"
  In1/1 -> Scope/2, If Action Subsystem/1(In1)  "Data"
  If/1 -> If Action Subsystem/Action
  In2/1 -> If/1, Scope/3  "Carry"

== system V1_DC_AC_PR_GF/Subsystem1/v2Low acquisition ==
  In1 : Inport
  In2 : Inport  Port=2
  If : If  IfExpression=u1 > 0.99  ShowElse=off
  If Action Subsystem : Subsystem  TreatAsAtomicUnit=on
  Scope : Scope  NumInputPorts=3
  v2Meas : Outport
  wires:
  If Action Subsystem/1(Out1) -> Scope/1, v2Meas/1  "Data_Carry"
  In1/1 -> Scope/2, If Action Subsystem/1(In1)  "Data"
  If/1 -> If Action Subsystem/Action
  In2/1 -> If/1, Scope/3  "Carry"

== system V1_DC_AC_PR_GF/Subsystem1/vHigh acquisition ==
  In1 : Inport
  In2 : Inport  Port=2
  If : If  IfExpression=u1 > 0.99  ShowElse=off
  If Action Subsystem : Subsystem  TreatAsAtomicUnit=on
  Scope : Scope  NumInputPorts=3
  vHMeas : Outport
  wires:
  If Action Subsystem/1(Out1) -> Scope/1, vHMeas/1  "Data_Carry"
  In1/1 -> Scope/2, If Action Subsystem/1(In1)  "Data"
  If/1 -> If Action Subsystem/Action
  In2/1 -> If/1, Scope/3  "Carry"

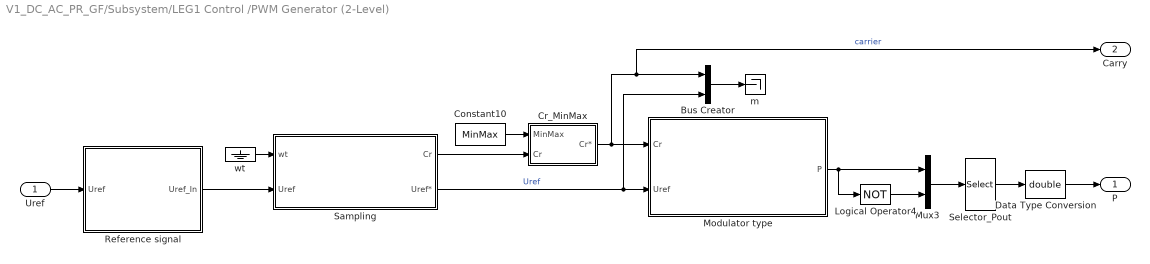
== system V1_DC_AC_PR_GF/Subsystem/LEG1 Control /PWM Generator (2-Level) ==
  Uref : Inport  PortDimensions=sps.UrefInport_PortDimensions  SampleTime=Ts
  Bus Creator : BusCreator  Inputs=2
  Constant10 : Constant  Value=MinMax
  Cr_MinMax : Subsystem
  Data Type Conversion : DataTypeConversion  OutDataTypeStr=double  SaturateOnIntegerOverflow=off  RndMeth=Floor
  Logical Operator4 : Logic  Operator=NOT
  Modulator type : Subsystem  BlockChoice=One_Three_PhaseBridge  Variant=on  VariantControlMode=label  LabelModeActiveChoice=OneThreePhaseBridge
  Mux3 : Mux  Inputs=2
  Reference signal : Subsystem  BlockChoice=InternalUref  Variant=on  VariantControlMode=label  LabelModeActiveChoice=External
  Sampling : Subsystem  BlockChoice=Unsync_NaturalSampling  Variant=on  VariantControlMode=label  LabelModeActiveChoice=UnsyncSymmetrical
  Selector_Pout : Selector  InputPortWidth=sps.SelectorPout_PortSize  IndexOptions=Index vector (dialog)  Indices=sps.SelectorPout_Index  OutputSizes=1
  m : Terminator
  wt : Ground
  P : Outport  SampleTime=Ts  VectorParamsAs1DForOutWhenUnconnected=off
  Carry : Outport  Port=2  SampleTime=Ts  VectorParamsAs1DForOutWhenUnconnected=off
  wires:
  wt/1 -> Sampling/1(wt)
  Reference signal/1(Uref_In) -> Sampling/2(Uref)
  Modulator type/1(P) -> Logical Operator4/1, Mux3/1
  Constant10/1 -> Cr_MinMax/1(MinMax)
  Uref/1 -> Reference signal/1(Uref)
  Data Type Conversion/1 -> P/1
  Logical Operator4/1 -> Mux3/2
  Mux3/1 -> Selector_Pout/1
  Selector_Pout/1 -> Data Type Conversion/1
  Cr_MinMax/1(Cr*) -> Carry/1, Bus Creator/1, Modulator type/1(Cr)  "carrier"
  Sampling/1(Cr) -> Cr_MinMax/2(Cr)
  Sampling/2(Uref*) -> Bus Creator/2, Modulator type/2(Uref)  "Uref"
  Bus Creator/1 -> m/1

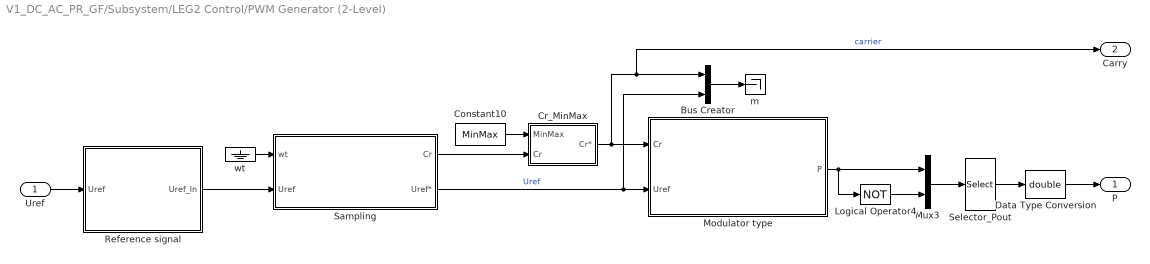
== system V1_DC_AC_PR_GF/Subsystem/LEG2 Control/PWM Generator (2-Level) ==
  Uref : Inport  PortDimensions=sps.UrefInport_PortDimensions  SampleTime=Ts
  Bus Creator : BusCreator  Inputs=2
  Constant10 : Constant  Value=MinMax
  Cr_MinMax : Subsystem
  Data Type Conversion : DataTypeConversion  OutDataTypeStr=double  SaturateOnIntegerOverflow=off  RndMeth=Floor
  Logical Operator4 : Logic  Operator=NOT
  Modulator type : Subsystem  BlockChoice=One_Three_PhaseBridge  Variant=on  VariantControlMode=label  LabelModeActiveChoice=OneThreePhaseBridge
  Mux3 : Mux  Inputs=2
  Reference signal : Subsystem  BlockChoice=InternalUref  Variant=on  VariantControlMode=label  LabelModeActiveChoice=External
  Sampling : Subsystem  BlockChoice=Unsync_NaturalSampling  Variant=on  VariantControlMode=label  LabelModeActiveChoice=UnsyncSymmetrical
  Selector_Pout : Selector  InputPortWidth=sps.SelectorPout_PortSize  IndexOptions=Index vector (dialog)  Indices=sps.SelectorPout_Index  OutputSizes=1
  m : Terminator
  wt : Ground
  P : Outport  SampleTime=Ts  VectorParamsAs1DForOutWhenUnconnected=off
  Carry : Outport  Port=2  SampleTime=Ts  VectorParamsAs1DForOutWhenUnconnected=off
  wires:
  Bus Creator/1 -> m/1
  Sampling/2(Uref*) -> Modulator type/2(Uref), Bus Creator/2  "Uref"
  Sampling/1(Cr) -> Cr_MinMax/2(Cr)
  Cr_MinMax/1(Cr*) -> Modulator type/1(Cr), Bus Creator/1, Carry/1  "carrier"
  Selector_Pout/1 -> Data Type Conversion/1
  Mux3/1 -> Selector_Pout/1
  Logical Operator4/1 -> Mux3/2
  Data Type Conversion/1 -> P/1
  Uref/1 -> Reference signal/1(Uref)
  Constant10/1 -> Cr_MinMax/1(MinMax)
  Modulator type/1(P) -> Mux3/1, Logical Operator4/1
  Reference signal/1(Uref_In) -> Sampling/2(Uref)
  wt/1 -> Sampling/1(wt)

== system V1_DC_AC_PR_GF/Subsystem1/i1Low acquisition/If Action Subsystem ==
  In1 : Inport
  Action Port : ActionPort  ActionPortLabel=if(u1 > 0.99)
  Out1 : Outport
  wires:
  In1/1 -> Out1/1

== system V1_DC_AC_PR_GF/Subsystem1/i2Low acquisition/If Action Subsystem ==
  In1 : Inport
  Action Port : ActionPort  ActionPortLabel=if(u1 > 0.99)
  Out1 : Outport
  wires:
  In1/1 -> Out1/1

== system V1_DC_AC_PR_GF/Subsystem1/iHigh acquisition/If Action Subsystem ==
  In1 : Inport
  Action Port : ActionPort  ActionPortLabel=if(u1 > 0.99)
  Out1 : Outport
  wires:
  In1/1 -> Out1/1

== system V1_DC_AC_PR_GF/Subsystem1/v1Low acquisition/If Action Subsystem ==
  In1 : Inport
  Action Port : ActionPort  ActionPortLabel=if(u1 > 0.99)
  Out1 : Outport
  wires:
  In1/1 -> Out1/1

== system V1_DC_AC_PR_GF/Subsystem1/v2Low acquisition/If Action Subsystem ==
  In1 : Inport
  Action Port : ActionPort  ActionPortLabel=if(u1 > 0.99)
  Out1 : Outport
  wires:
  In1/1 -> Out1/1

== system V1_DC_AC_PR_GF/Subsystem1/vHigh acquisition/If Action Subsystem ==
  In1 : Inport
  Action Port : ActionPort  ActionPortLabel=if(u1 > 0.99)
  Out1 : Outport
  wires:
  In1/1 -> Out1/1

== system V1_DC_AC_PR_GF/Subsystem/LEG1 Control /PWM Generator (2-Level)/Cr_MinMax ==
  MinMax : Inport
  Cr : Inport  Port=2
  Add3 : Sum  Inputs=-+
  Add4 : Sum  Inputs=+++
  Demux : Demux  Outputs=2
  Gain1 : Gain  Gain=0.5
  MUL1 : Product  Inputs=**
  Cr* : Outport  VectorParamsAs1DForOutWhenUnconnected=off
  wires:
  Add3/1 -> Gain1/1
  MinMax/1 -> Demux/1
  Demux/1 -> Add4/1, Add3/1
  Demux/2 -> Add3/2
  Gain1/1 -> Add4/3, MUL1/2
  Cr/1 -> MUL1/1
  Add4/1 -> Cr*/1
  MUL1/1 -> Add4/2

== system V1_DC_AC_PR_GF/Subsystem/LEG1 Control /PWM Generator (2-Level)/Modulator type ==
  Cr : Inport
  Uref : Inport  Port=2
  Full Bridge Bipolar : Subsystem  VariantControl=FullBridgeBipolar
  Full Bridge Unipolar : Subsystem  VariantControl=FullBridgeUnipolar
  One Three Phase Bridge : Subsystem  VariantControl=OneThreePhaseBridge
  P : Outport  VectorParamsAs1DForOutWhenUnconnected=off

== system V1_DC_AC_PR_GF/Subsystem/LEG1 Control /PWM Generator (2-Level)/Reference signal ==
  Uref : Inport
  External : Subsystem  VariantControl=External
  Internal : Subsystem  VariantControl=Internal
  Uref_In : Outport  VectorParamsAs1DForOutWhenUnconnected=off

== system V1_DC_AC_PR_GF/Subsystem/LEG1 Control /PWM Generator (2-Level)/Sampling ==
  wt : Inport
  Uref : Inport  Port=2
  Sync Asymmetrical : Subsystem  VariantControl=SyncAsymmetrical
  Sync Natural : Subsystem  VariantControl=SyncNatural
  Sync Symmetrical : Subsystem  VariantControl=SyncSymmetrical
  Unsync Asymmetrical : Subsystem  VariantControl=UnsyncAsymmetrical
  Unsync Natural : Subsystem  VariantControl=UnsyncNatural
  Unsync Symmetrical : Subsystem  VariantControl=UnsyncSymmetrical
  Cr : Outport  VectorParamsAs1DForOutWhenUnconnected=off
  Uref* : Outport  Port=2  VectorParamsAs1DForOutWhenUnconnected=off

== system V1_DC_AC_PR_GF/Subsystem/LEG2 Control/PWM Generator (2-Level)/Cr_MinMax ==
  MinMax : Inport
  Cr : Inport  Port=2
  Add3 : Sum  Inputs=-+
  Add4 : Sum  Inputs=+++
  Demux : Demux  Outputs=2
  Gain1 : Gain  Gain=0.5
  MUL1 : Product  Inputs=**
  Cr* : Outport  VectorParamsAs1DForOutWhenUnconnected=off
  wires:
  MUL1/1 -> Add4/2
  Add4/1 -> Cr*/1
  Cr/1 -> MUL1/1
  Gain1/1 -> MUL1/2, Add4/3
  Demux/2 -> Add3/2
  Demux/1 -> Add3/1, Add4/1
  MinMax/1 -> Demux/1
  Add3/1 -> Gain1/1

== system V1_DC_AC_PR_GF/Subsystem/LEG2 Control/PWM Generator (2-Level)/Modulator type ==
  Cr : Inport
  Uref : Inport  Port=2
  Full Bridge Bipolar : Subsystem  VariantControl=FullBridgeBipolar
  Full Bridge Unipolar : Subsystem  VariantControl=FullBridgeUnipolar
  One Three Phase Bridge : Subsystem  VariantControl=OneThreePhaseBridge
  P : Outport  VectorParamsAs1DForOutWhenUnconnected=off

== system V1_DC_AC_PR_GF/Subsystem/LEG2 Control/PWM Generator (2-Level)/Reference signal ==
  Uref : Inport
  External : Subsystem  VariantControl=External
  Internal : Subsystem  VariantControl=Internal
  Uref_In : Outport  VectorParamsAs1DForOutWhenUnconnected=off

== system V1_DC_AC_PR_GF/Subsystem/LEG2 Control/PWM Generator (2-Level)/Sampling ==
  wt : Inport
  Uref : Inport  Port=2
  Sync Asymmetrical : Subsystem  VariantControl=SyncAsymmetrical
  Sync Natural : Subsystem  VariantControl=SyncNatural
  Sync Symmetrical : Subsystem  VariantControl=SyncSymmetrical
  Unsync Asymmetrical : Subsystem  VariantControl=UnsyncAsymmetrical
  Unsync Natural : Subsystem  VariantControl=UnsyncNatural
  Unsync Symmetrical : Subsystem  VariantControl=UnsyncSymmetrical
  Cr : Outport  VectorParamsAs1DForOutWhenUnconnected=off
  Uref* : Outport  Port=2  VectorParamsAs1DForOutWhenUnconnected=off

== system V1_DC_AC_PR_GF/Subsystem/LEG1 Control /PWM Generator (2-Level)/Modulator type/Full Bridge Bipolar ==
  Cr : Inport
  Uref : Inport  Port=2
  Logical Operator : Logic  Operator=NOT  AllPortsSameDT=off  OutDataTypeStr=boolean
  Mux1 : Mux  Inputs=2
  Relational Operator2 : RelationalOperator  OutDataTypeStr=boolean
  Selector_FullBridgeIn : Selector  InputPortWidth=sps.SelectorFullBridgeIn_PortSize  IndexOptions=Index vector (dialog)  Indices=[1]  OutputSizes=1
  Selector_FullBridgeOut1 : Selector  InputPortWidth=2  IndexOptions=Index vector (dialog)  Indices=sps.SelectorFullBridgeOut_Index  OutputSizes=1
  P : Outport  SampleTime=Ts  VectorParamsAs1DForOutWhenUnconnected=off
  wires:
  Uref/1 -> Selector_FullBridgeIn/1
  Selector_FullBridgeIn/1 -> Relational Operator2/1
  Selector_FullBridgeOut1/1 -> P/1
  Cr/1 -> Relational Operator2/2
  Mux1/1 -> Selector_FullBridgeOut1/1
  Relational Operator2/1 -> Mux1/1, Logical Operator/1
  Logical Operator/1 -> Mux1/2

== system V1_DC_AC_PR_GF/Subsystem/LEG1 Control /PWM Generator (2-Level)/Modulator type/Full Bridge Unipolar ==
  Cr : Inport
  Uref : Inport  Port=2
  Gain : Gain  Gain=-1
  Mux : Mux  Inputs=2
  Relational Operator1 : RelationalOperator  OutDataTypeStr=boolean
  Relational Operator3 : RelationalOperator  OutDataTypeStr=boolean
  Selector_FullBridgeIn : Selector  InputPortWidth=sps.SelectorFullBridgeIn_PortSize  IndexOptions=Index vector (dialog)  Indices=[1]  OutputSizes=1
  Selector_FullBridgeOut : Selector  InputPortWidth=2  IndexOptions=Index vector (dialog)  Indices=sps.SelectorFullBridgeOut_Index  OutputSizes=1
  P : Outport  SampleTime=Ts  VectorParamsAs1DForOutWhenUnconnected=off
  wires:
  Uref/1 -> Selector_FullBridgeIn/1
  Selector_FullBridgeIn/1 -> Relational Operator1/1, Gain/1
  Selector_FullBridgeOut/1 -> P/1
  Gain/1 -> Relational Operator3/1
  Relational Operator1/1 -> Mux/1
  Relational Operator3/1 -> Mux/2
  Mux/1 -> Selector_FullBridgeOut/1
  Cr/1 -> Relational Operator3/2, Relational Operator1/2

== system V1_DC_AC_PR_GF/Subsystem/LEG1 Control /PWM Generator (2-Level)/Modulator type/One Three Phase Bridge ==
  Cr : Inport
  Uref : Inport  Port=2
  Relational Operator2 : RelationalOperator  OutDataTypeStr=boolean
  Selector_HalfBridgeOut : Selector  InputPortWidth=sps.SelectorHalfBridgeOut_PortSize  IndexOptions=Index vector (dialog)  Indices=sps.SelectorHalfBridgeOut_Index  OutputSizes=1
  P : Outport  PortDimensions=sps.SelectorHalfBridgeOut_PortSize  SampleTime=Ts  VectorParamsAs1DForOutWhenUnconnected=off
  wires:
  Uref/1 -> Relational Operator2/1
  Selector_HalfBridgeOut/1 -> P/1
  Cr/1 -> Relational Operator2/2
  Relational Operator2/1 -> Selector_HalfBridgeOut/1

== system V1_DC_AC_PR_GF/Subsystem/LEG1 Control /PWM Generator (2-Level)/Reference signal/External ==
  Uref : Inport  PortDimensions=sps.UrefInport_PortDimensions  SampleTime=Ts
  Uref_In : Outport  VectorParamsAs1DForOutWhenUnconnected=off
  wires:
  Uref/1 -> Uref_In/1

== system V1_DC_AC_PR_GF/Subsystem/LEG1 Control /PWM Generator (2-Level)/Reference signal/Internal ==
  Uref : Inport  PortDimensions=sps.UrefInport_PortDimensions  SampleTime=Ts
  Sine Wave : Sin  Amplitude=sps.m  Frequency=sps.Freq  Phase=sps.SinWave_Phase  SampleTime=Ts
  end : Terminator
  Uref_In : Outport  VectorParamsAs1DForOutWhenUnconnected=off
  wires:
  Sine Wave/1 -> Uref_In/1
  Uref/1 -> end/1

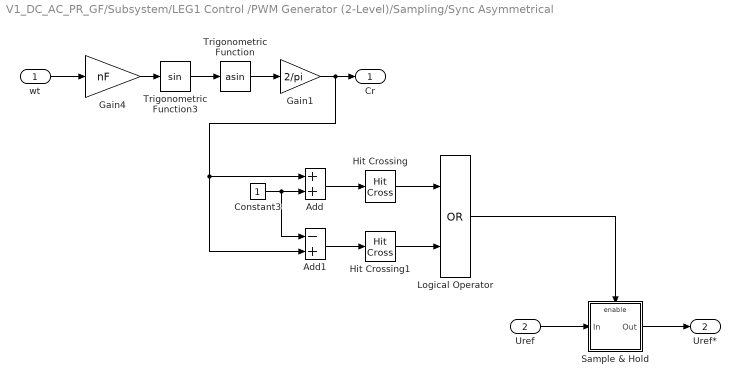
== system V1_DC_AC_PR_GF/Subsystem/LEG1 Control /PWM Generator (2-Level)/Sampling/Sync Asymmetrical ==
  wt : Inport  Interpolate=off
  Uref : Inport  Port=2  Interpolate=off
  Add : Sum
  Add1 : Sum  Inputs=-+
  Constant3 : Constant
  Gain1 : Gain  Gain=2/pi  SaturateOnIntegerOverflow=on  OutDataTypeStr=Inherit: Same as input  ParamDataTypeStr=Inherit: Same as input
  Gain4 : Gain  Gain=nF  SaturateOnIntegerOverflow=on  OutDataTypeStr=Inherit: Same as input  ParamDataTypeStr=Inherit: Same as input
  Hit Crossing : HitCross  HitCrossingOffset=1e-9  HitCrossingDirection=falling
  Hit Crossing1 : HitCross  HitCrossingOffset=-1e-9  HitCrossingDirection=rising
  Logical Operator : Logic  Operator=OR  AllPortsSameDT=off  OutDataTypeStr=boolean
  Sample & Hold : Subsystem
  Trigonometric Function : Trigonometry  Operator=asin
  Trigonometric Function3 : Trigonometry
  Cr : Outport  VectorParamsAs1DForOutWhenUnconnected=off
  Uref* : Outport  Port=2  VectorParamsAs1DForOutWhenUnconnected=off
  wires:
  wt/1 -> Gain4/1
  Gain1/1 -> Cr/1, Add1/2, Add/1
  Trigonometric Function/1 -> Gain1/1
  Trigonometric Function3/1 -> Trigonometric Function/1
  Gain4/1 -> Trigonometric Function3/1
  Constant3/1 -> Add/2, Add1/1
  Add/1 -> Hit Crossing/1
  Add1/1 -> Hit Crossing1/1
  Uref/1 -> Sample & Hold/1(In)
  Sample & Hold/1(Out) -> Uref*/1
  Logical Operator/1 -> Sample & Hold/Enable
  Hit Crossing/1 -> Logical Operator/1
  Hit Crossing1/1 -> Logical Operator/2

== system V1_DC_AC_PR_GF/Subsystem/LEG1 Control /PWM Generator (2-Level)/Sampling/Sync Natural ==
  wt : Inport
  Uref : Inport  Port=2
  Sync_NaturalSampling : Subsystem
  Cr : Outport  VectorParamsAs1DForOutWhenUnconnected=off
  Uref* : Outport  Port=2  VectorParamsAs1DForOutWhenUnconnected=off
  wires:
  Uref/1 -> Sync_NaturalSampling/1(Uref)
  wt/1 -> Sync_NaturalSampling/2(wt)
  Sync_NaturalSampling/1(Uref*) -> Uref*/1
  Sync_NaturalSampling/2(Cr) -> Cr/1

== system V1_DC_AC_PR_GF/Subsystem/LEG1 Control /PWM Generator (2-Level)/Sampling/Sync Symmetrical ==
  wt : Inport
  Uref : Inport  Port=2
  Sync_SymmetricalSampling : Subsystem
  Cr : Outport  VectorParamsAs1DForOutWhenUnconnected=off
  Uref* : Outport  Port=2  VectorParamsAs1DForOutWhenUnconnected=off
  wires:
  Uref/1 -> Sync_SymmetricalSampling/1(Uref)
  wt/1 -> Sync_SymmetricalSampling/2(wt)
  Sync_SymmetricalSampling/1(Uref*) -> Uref*/1
  Sync_SymmetricalSampling/2(Cr) -> Cr/1

== system V1_DC_AC_PR_GF/Subsystem/LEG1 Control /PWM Generator (2-Level)/Sampling/Unsync Asymmetrical ==
  wt : Inport
  Uref : Inport  Port=2
  Unsync_AsymmetricalSampling : Subsystem
  term1 : Terminator
  Cr : Outport  VectorParamsAs1DForOutWhenUnconnected=off
  Uref* : Outport  Port=2  VectorParamsAs1DForOutWhenUnconnected=off
  wires:
  Uref/1 -> Unsync_AsymmetricalSampling/1(Uref)
  Unsync_AsymmetricalSampling/1(Uref*) -> Uref*/1
  Unsync_AsymmetricalSampling/2(Cr) -> Cr/1
  wt/1 -> term1/1

== system V1_DC_AC_PR_GF/Subsystem/LEG1 Control /PWM Generator (2-Level)/Sampling/Unsync Natural ==
  wt : Inport
  Uref : Inport  Port=2
  Unsync_NaturalSampling : Subsystem
  term1 : Terminator
  Cr : Outport  VectorParamsAs1DForOutWhenUnconnected=off
  Uref* : Outport  Port=2  VectorParamsAs1DForOutWhenUnconnected=off
  wires:
  Uref/1 -> Unsync_NaturalSampling/1(Uref)
  Unsync_NaturalSampling/1(Uref*) -> Uref*/1
  Unsync_NaturalSampling/2(Cr) -> Cr/1
  wt/1 -> term1/1

== system V1_DC_AC_PR_GF/Subsystem/LEG1 Control /PWM Generator (2-Level)/Sampling/Unsync Symmetrical ==
  wt : Inport
  Uref : Inport  Port=2
  Unsync_SymmetricalSampling : Subsystem
  term1 : Terminator
  Cr : Outport  VectorParamsAs1DForOutWhenUnconnected=off
  Uref* : Outport  Port=2  VectorParamsAs1DForOutWhenUnconnected=off
  wires:
  Uref/1 -> Unsync_SymmetricalSampling/1(Uref)
  Unsync_SymmetricalSampling/1(Uref*) -> Uref*/1
  Unsync_SymmetricalSampling/2(Cr) -> Cr/1
  wt/1 -> term1/1

== system V1_DC_AC_PR_GF/Subsystem/LEG2 Control/PWM Generator (2-Level)/Modulator type/Full Bridge Bipolar ==
  Cr : Inport
  Uref : Inport  Port=2
  Logical Operator : Logic  Operator=NOT  AllPortsSameDT=off  OutDataTypeStr=boolean
  Mux1 : Mux  Inputs=2
  Relational Operator2 : RelationalOperator  OutDataTypeStr=boolean
  Selector_FullBridgeIn : Selector  InputPortWidth=sps.SelectorFullBridgeIn_PortSize  IndexOptions=Index vector (dialog)  Indices=[1]  OutputSizes=1
  Selector_FullBridgeOut1 : Selector  InputPortWidth=2  IndexOptions=Index vector (dialog)  Indices=sps.SelectorFullBridgeOut_Index  OutputSizes=1
  P : Outport  SampleTime=Ts  VectorParamsAs1DForOutWhenUnconnected=off
  wires:
  Logical Operator/1 -> Mux1/2
  Relational Operator2/1 -> Logical Operator/1, Mux1/1
  Mux1/1 -> Selector_FullBridgeOut1/1
  Cr/1 -> Relational Operator2/2
  Selector_FullBridgeOut1/1 -> P/1
  Selector_FullBridgeIn/1 -> Relational Operator2/1
  Uref/1 -> Selector_FullBridgeIn/1

== system V1_DC_AC_PR_GF/Subsystem/LEG2 Control/PWM Generator (2-Level)/Modulator type/Full Bridge Unipolar ==
  Cr : Inport
  Uref : Inport  Port=2
  Gain : Gain  Gain=-1
  Mux : Mux  Inputs=2
  Relational Operator1 : RelationalOperator  OutDataTypeStr=boolean
  Relational Operator3 : RelationalOperator  OutDataTypeStr=boolean
  Selector_FullBridgeIn : Selector  InputPortWidth=sps.SelectorFullBridgeIn_PortSize  IndexOptions=Index vector (dialog)  Indices=[1]  OutputSizes=1
  Selector_FullBridgeOut : Selector  InputPortWidth=2  IndexOptions=Index vector (dialog)  Indices=sps.SelectorFullBridgeOut_Index  OutputSizes=1
  P : Outport  SampleTime=Ts  VectorParamsAs1DForOutWhenUnconnected=off
  wires:
  Cr/1 -> Relational Operator1/2, Relational Operator3/2
  Mux/1 -> Selector_FullBridgeOut/1
  Relational Operator3/1 -> Mux/2
  Relational Operator1/1 -> Mux/1
  Gain/1 -> Relational Operator3/1
  Selector_FullBridgeOut/1 -> P/1
  Selector_FullBridgeIn/1 -> Gain/1, Relational Operator1/1
  Uref/1 -> Selector_FullBridgeIn/1
